simulink model "untitled"  (R2014a)
settings: Solver=ode45  StartTime=0.0  StopTime=10.0  RelTol=1e-3
libraries: neural x25
(part 2 of 4)

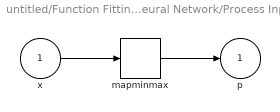
== system untitled/Function Fitting Neural Network/Process Input 1 ==
  x : Inport  PortDimensions=4800
      mask Display: e = 0.06;c1 = [120 230 180]/255;c2 = ([120 230 180]+0)/(256+128);c3 = ([120 230 180]+128)/(256+128);patch([0 1 1 0],[0 0 1 1],c1);patch([0 1 1 1-e 1-e 0+e],[0 0 1 1-e 0+e 0+e],c2);patch([0 0 1 1-e 0+e 0+e],[0 1 1 1-e 1-e 0+e],c3);plot([0 1 1 0 0],[0 0 1 1 0]);
  mapminmax : neural/Processing Functions/mapminmax  xmin=[11;15;11;8;12;9;8;13;9;4;13;9;7;14;9;8;16;13;9;13;13;10;12;10;9;8;0;7;11;10;9;8;14;7;11;4;7;11;10;4;10;7;1;11;13;7;13;17;2;10;19;0;2;0;6;8;12;6;10;13;3;12;14;5;13;10;2;11;9;4;8;14;0;11;12;8;13;33;6;7;13;8;12;51;6;12;46;0;0;0;1;14;62;0;8;26;4;8;52;4;7;7;3;10;8;8;9;26;6;10;14;0;5;4;4;7;31;1;7;10;3;5;12;0;6;3;2;8;4;0;14;15;1;10;62;5;9;16;0;7;69;0;7;65;0;7;97;4;10;31;6;11;31;3;10;8;2;9;67;3;11;74;1;9;68;0;5;66;0;7;69;4;11;36;4;7;94;1;9;79;0;7;36;0;1;38;2;8;45;0;4;37;1;6;73;3;7;81;4;8;36;5;9;21;0;5;49;1;1;25;2;6;32;0;7;42;1;6;39;3;9;70;3;6;64;2;3;111;4;9;89;6;9;92;4;8;26;0;7;13;1;6;29;0;8;16;0;6;70;0;7;91;0;8;90;0;8;42;1;7;15;0;3;19;0;5;47;4;9;88;0;9;89;0;7;94;0;5;54;0;4;22;1;5;74;0;3;26;0;3;31;0;5;101;0;5;87;0;1;10;0;7;53;0;8;86;1;8;87;0;1;97;0;4;68;2;0;83;0;5;98;0;7;65;1;8;56;0;6;9;0;8;73;0;1;106;0;4;108;0;6;92;0;0;113;0;8;93;0;6;77;1;5;79;2;7;40;0;5;27;0;3;74;0;3;101;0;3;42;0;2;24;0;7;67;0;7;92;1;8;97;0;1;82;0;0;79;0;8;59;0;7;51;1;7;26;2;6;86;1;7;84;2;7;90;0;6;96;0;5;110;1;7;88;0;0;19;0;6;35;0;6;31;1;4;82;0;4;31;0;0;60;0;4;34;3;8;78;2;4;81;2;6;18;3;5;75;2;6;41;2;8;75;0;5;35;0;2;57;2;8;89;0;5;94;0;6;86;0;5;84;0;8;102;1;5;69;0;4;49;0;4;49;1;5;69;0;8;102;0;5;84;0;6;86;0;5;94;2;8;89;0;2;57;0;5;35;2;8;75;2;6;41;3;5;75;2;6;18;2;4;81;3;8;78;0;4;34;0;0;60;0;4;31;1;4;82;0;6;31;0;6;35;0;0;19;1;7;88;0;5;110;0;6;96;2;7;90;1;7;84;2;6;86;1;7;26;0;7;51;0;8;59;0;0;79;0;1;82;1;8;97;0;7;92;0;7;67;0;2;24;0;3;42;0;3;101;0;3;74;0;5;27;2;7;40;1;5;79;0;6;77;0;8;93;0;0;113;0;6;92;0;4;108;0;1;106;0;8;73;0;6;9;1;8;56;0;7;65;0;5;98;2;0;83;0;4;68;0;1;97;1;8;87;0;8;86;0;7;53;0;1;10;0;5;87;0;5;101;0;3;31;0;3;26;1;5;74;0;4;22;0;5;54;0;7;94;0;9;89;4;9;88;0;5;47;0;3;19;1;7;15;0;8;42;0;8;90;0;7;91;0;6;70;0;8;16;1;6;29;0;7;13;4;8;26;6;9;92;4;9;89;2;3;111;3;6;64;3;9;70;1;6;39;0;7;42;2;6;32;1;1;25;0;5;49;5;9;21;4;8;36;3;7;81;1;6;73;0;4;37;2;8;45;0;1;38;0;7;36;1;9;79;4;7;94;4;11;36;0;7;69;0;5;66;1;9;68;3;11;74;2;9;67;3;10;8;6;11;31;4;10;31;0;7;97;0;7;65;0;7;69;5;9;16;1;10;62;0;14;15;2;8;4;0;6;3;3;5;12;1;7;10;4;7;31;0;5;4;6;10;14;8;9;26;3;10;8;4;7;7;4;8;52;0;8;26;1;14;62;0;0;0;6;12;46;8;12;51;6;7;13;8;13;33;0;11;12;4;8;14;2;11;9;5;13;10;3;12;14;6;10;13;6;8;12;0;2;0;2;10;19;7;13;17;1;11;13;4;10;7;7;11;10;7;11;4;9;8;14;7;11;10;9;8;0;10;12;10;9;13;13;8;16;13;7;14;9;4;13;9;8;13;9;8;12;9;11;15;11;6;11;8;7;13;3;6;10;9;7;13;8;8;13;8;8;10;7;8;0;0;10;12;7;9;14;13;5;7;5;8;7;3;6;14;9;10;15;16;0;6;1;9;15;8;2;11;12;9;8;14;0;4;2;8;9;8;8;12;14;6;13;6;8;13;14;0;2;0;2;10;19;3;13;51;7;13;9;2;11;47;7;8;69;7;12;53;0;1;0;6;10;50;0;5;3;6;12;43;6;13;13;4;9;8;6;11;51;0;4;2;7;11;24;7;14;84;0;7;5;6;9;25;5;11;18;7;10;10;4;8;6;3;10;52;7;11;44;7;9;43;3;7;43;6;10;58;1;9;87;6;10;89;4;11;14;4;11;73;0;7;84;2;11;53;0;6;78;0;11;62;0;6;1;5;9;80;4;9;72;2;10;48;2;6;23;0;8;24;1;9;70;1;9;62;4;11;73;5;8;49;6;10;59;3;9;15;3;4;23;3;7;10;0;1;33;1;8;25;0;1;80;3;5;94;2;11;116;5;9;88;6;9;59;5;5;19;0;6;23;0;0;13;0;1;0;2;9;9;2;9;53;0;9;19;1;8;12;4;10;17;0;0;78;1;6;41;3;6;37;0;6;78;3;1;47;0;4;64;1;5;97;2;7;51;0;6;11;1;7;43;0;7;40;0;5;14;0;0;82;0;9;89;1;7;36;2;6;15;0;2;83;0;7;95;3;0;49;1;5;63;0;0;95;2;5;113;0;7;115;2;9;44;0;2;23;0;0;75;0;3;98;0;6;106;1;0;90;3;6;93;3;7;37;5;8;35;0;3;51;0;4;39;2;5;15;2;7;43;0;4;77;1;6;92;0;1;89;1;6;96;0;6;79;2;4;121;2;4;125;0;8;96;2;6;99;2;8;23;3;6;50;3;7;93;0;0;64;0;5;14;0;1;66;0;7;100;3;6;50;2;5;13;2;1;23;4;10;46;0;7;62;0;7;42;0;4;3;2;8;39;0;0;0;3;9;75;2;9;16;2;8;59;0;6;81;0;0;75;3;7;68;2;4;119;1;8;124;0;9;86;0;7;85;1;8;60;2;7;70;2;7;70;1;8;60;0;7;85;0;9;86;1;8;124;2;4;119;3;7;68;0;0;75;0;6;81;2;8;59;2;9;16;3;9;75;0;0;0;2;8;39;0;4;3;0;7;42;0;7;62;4;10;46;2;1;23;2;5;13;3;6;50;0;7;100;0;1;66;0;5;14;0;0;64;3;7;93;3;6;50;2;8;23;2;6;99;0;8;96;2;4;125;2;4;121;0;6;79;1;6;96;0;1;89;1;6;92;0;4;77;2;7;43;2;5;15;0;4;39;0;3;51;5;8;35;3;7;37;3;6;93;1;0;90;0;6;106;0;3;98;0;0;75;0;2;23;2;9;44;0;7;115;2;5;113;0;0;95;1;5;63;3;0;49;0;7;95;0;2;83;2;6;15;1;7;36;0;9;89;0;0;82;0;5;14;0;7;40;1;7;43;0;6;11;2;7;51;1;5;97;0;4;64;3;1;47;0;6;78;3;6;37;1;6;41;0;0;78;4;10;17;1;8;12;0;9;19;2;9;53;2;9;9;0;1;0;0;0 ...(+7521 chars)]  xmax=[198;196;195;226;210;206;250;229;225;236;234;230;237;236;232;233;232;228;223;222;218;235;234;230;227;223;221;209;206;202;232;229;225;220;219;215;206;207;205;232;236;231;240;244;239;217;219;214;234;236;231;231;229;228;235;233;232;222;220;219;239;240;236;237;238;234;203;204;200;189;190;186;223;224;220;217;218;214;242;246;241;240;244;239;239;243;238;234;238;233;240;244;239;232;235;230;244;244;241;234;238;233;241;242;238;215;216;212;236;240;235;240;241;237;235;236;232;215;216;212;231;232;230;238;244;239;243;244;240;238;239;235;241;242;238;242;243;241;233;234;230;217;218;214;240;244;239;234;238;233;229;230;226;240;241;237;239;240;236;232;233;229;211;212;213;218;222;217;205;205;205;211;212;210;215;216;214;212;213;209;239;243;238;244;245;241;239;240;236;243;244;240;234;237;236;237;240;238;238;239;235;238;239;235;243;244;240;241;242;240;243;244;240;238;239;245;240;241;237;239;240;238;223;224;240;240;241;237;234;235;231;230;231;228;239;240;236;235;236;232;236;237;233;243;241;237;243;246;244;227;228;226;218;219;217;233;239;234;241;247;242;235;241;236;240;245;247;197;197;218;181;185;199;241;246;245;236;242;241;249;248;244;230;238;237;232;240;239;234;244;244;208;216;216;189;188;241;192;196;209;204;206;237;180;184;216;179;185;239;189;193;228;185;201;239;179;186;221;232;233;229;203;204;224;204;210;213;205;205;222;179;184;218;184;190;237;188;188;218;191;198;221;189;191;239;217;220;234;214;217;240;217;216;227;228;225;226;209;210;223;218;214;213;230;224;221;229;225;222;204;203;226;207;207;238;210;209;229;221;219;243;203;199;248;192;185;207;221;215;231;212;207;239;219;216;236;181;187;214;215;214;223;215;212;232;228;225;239;193;200;235;183;189;228;211;216;245;208;212;207;214;211;232;224;223;220;190;189;231;230;230;230;230;224;225;225;218;227;232;239;250;231;240;227;215;215;217;210;207;244;213;219;241;225;219;233;226;222;219;213;211;211;219;218;215;208;206;219;231;238;234;244;251;246;212;219;225;221;223;222;221;223;222;212;219;225;244;251;246;231;238;234;208;206;219;219;218;215;213;211;211;226;222;219;225;219;233;213;219;241;210;207;244;215;215;217;231;240;227;232;239;250;225;218;227;230;224;225;230;230;230;190;189;231;224;223;220;214;211;232;208;212;207;211;216;245;183;189;228;193;200;235;228;225;239;215;212;232;215;214;223;181;187;214;219;216;236;212;207;239;221;215;231;192;185;207;203;199;248;221;219;243;210;209;229;207;207;238;204;203;226;229;225;222;230;224;221;218;214;213;209;210;223;228;225;226;217;216;227;214;217;240;217;220;234;189;191;239;191;198;221;188;188;218;184;190;237;179;184;218;205;205;222;204;210;213;203;204;224;232;233;229;179;186;221;185;201;239;189;193;228;179;185;239;180;184;216;204;206;237;192;196;209;189;188;241;208;216;216;234;244;244;232;240;239;230;238;237;249;248;244;236;242;241;241;246;245;181;185;199;197;197;218;240;245;247;235;241;236;241;247;242;233;239;234;218;219;217;227;228;226;243;246;244;243;241;237;236;237;233;235;236;232;239;240;236;230;231;228;234;235;231;240;241;237;223;224;240;239;240;238;240;241;237;238;239;245;243;244;240;241;242;240;243;244;240;238;239;235;238;239;235;237;240;238;234;237;236;243;244;240;239;240;236;244;245;241;239;243;238;212;213;209;215;216;214;211;212;210;205;205;205;218;222;217;211;212;213;232;233;229;239;240;236;240;241;237;229;230;226;234;238;233;240;244;239;217;218;214;233;234;230;242;243;241;241;242;238;238;239;235;243;244;240;238;244;239;231;232;230;215;216;212;235;236;232;240;241;237;236;240;235;215;216;212;241;242;238;234;238;233;244;244;241;232;235;230;240;244;239;234;238;233;239;243;238;240;244;239;242;246;241;217;218;214;223;224;220;189;190;186;203;204;200;237;238;234;239;240;236;222;220;219;235;233;232;231;229;228;234;236;231;217;219;214;240;244;239;232;236;231;206;207;205;220;219;215;232;229;225;209;206;202;227;223;221;235;234;230;223;222;218;233;232;228;237;236;232;236;234;230;250;229;225;226;210;206;198;196;195;255;238;237;240;241;239;239;240;238;232;233;231;211;217;212;239;245;240;245;246;242;236;236;232;239;240;238;245;246;244;237;238;236;234;233;229;222;221;217 ...(+15204 chars)]  ymin=-1  ymax=1
  p : Outport  PortDimensions=4800
      mask Display: e = 0.06;c1 = [120 230 180]/255;c2 = ([120 230 180]+0)/(256+128);c3 = ([120 230 180]+128)/(256+128);patch([0 1 1 0],[0 0 1 1],c1);patch([0 1 1 1-e 1-e 0+e],[0 0 1 1-e 0+e 0+e],c2);patch([0 0 1 1-e 0+e 0+e],[0 1 1 1-e 1-e 0+e],c3);plot([0 1 1 0 0],[0 0 1 1 0]);
  wires:
  x/1 -> mapminmax/1
  mapminmax/1 -> p/1

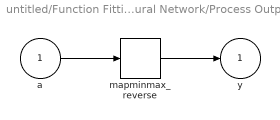
== system untitled/Function Fitting Neural Network/Process Output 1 ==
  a : Inport  PortDimensions=1
      mask Display: e = 0.06;c1 = [120 230 180]/255;c2 = ([120 230 180]+0)/(256+128);c3 = ([120 230 180]+128)/(256+128);patch([0 1 1 0],[0 0 1 1],c1);patch([0 1 1 1-e 1-e 0+e],[0 0 1 1-e 0+e 0+e],c2);patch([0 0 1 1-e 0+e 0+e],[0 1 1 1-e 1-e 0+e],c3);plot([0 1 1 0 0],[0 0 1 1 0]);
  mapminmax_reverse : neural/Processing Functions/mapminmax_reverse  xmin=5  xmax=314  ymin=-1  ymax=1
  y : Outport  PortDimensions=1
      mask Display: e = 0.06;c1 = [120 230 180]/255;c2 = ([120 230 180]+0)/(256+128);c3 = ([120 230 180]+128)/(256+128);patch([0 1 1 0],[0 0 1 1],c1);patch([0 1 1 1-e 1-e 0+e],[0 0 1 1-e 0+e 0+e],c2);patch([0 0 1 1-e 0+e 0+e],[0 1 1 1-e 1-e 0+e],c3);plot([0 1 1 0 0],[0 0 1 1 0]);
  wires:
  a/1 -> mapminmax_reverse/1
  mapminmax_reverse/1 -> y/1

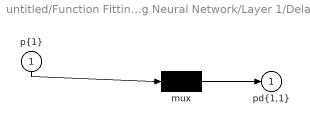
== system untitled/Function Fitting Neural Network/Layer 1/Delays 1 ==
  "p{1}" : Inport  PortDimensions=4800
      mask Display: e = 0.06;c1 = [120 230 180]/255;c2 = ([120 230 180]+0)/(256+128);c3 = ([120 230 180]+128)/(256+128);patch([0 1 1 0],[0 0 1 1],c1);patch([0 1 1 1-e 1-e 0+e],[0 0 1 1-e 0+e 0+e],c2);patch([0 0 1 1-e 0+e 0+e],[0 1 1 1-e 1-e 0+e],c3);plot([0 1 1 0 0],[0 0 1 1 0]);
  mux : Mux  Inputs=1
      mask Display: e = 0.06;c1 = [120 150 230]/255;c2 = ([120 150 230]+0)/383;c3 = ([120 150 230]+128)/383;patch([0 1 1 0],[0 0 1 1],c1);patch([0 1 1 1-e 1-e 0+e],[0 0 1 1-e 0+e 0+e],c2);patch([0 0 1 1-e 0+e 0+e],[0 1 1 1-e 1-e 0+e],c3);plot([0 1 1 0 0],[0 0 1 1 0]);disp('Mux')
  "pd{1,1}" : Outport
      mask Display: e = 0.06;c1 = [120 230 180]/255;c2 = ([120 230 180]+0)/(256+128);c3 = ([120 230 180]+128)/(256+128);patch([0 1 1 0],[0 0 1 1],c1);patch([0 1 1 1-e 1-e 0+e],[0 0 1 1-e 0+e 0+e],c2);patch([0 0 1 1-e 0+e 0+e],[0 1 1 1-e 1-e 0+e],c3);plot([0 1 1 0 0],[0 0 1 1 0]);
  wires:
  "p{1}"/1 -> mux/1
  mux/1 -> "pd{1,1}"/1
